simulink model "Ejercicio_Valvulas_simuslx"  (R2021a)
settings: Solver=VariableStepAuto  StartTime=0.0  StopTime=20  RelTol=1e-3
values from neighbouring files (symbols this model uses):
  K = [p1-a1 p2-a2] * Wrm * inv(Wr)    [Controlabilidad.m]    (also in Ejemplo_filminas.m; Ejercicio_Inestable.m = [p1 - a1, p2 - a2] * Wrm * inv(Wr); Ejercicio_Valvulas.m = Ka(1:order(P)); realimentacion_ee.m = acker(A, B, [-10 -10]))
  ue = x3e    [Ejercicio_Valvulas.m]
  xe = [x1e; x2e; x3e]    [Ejercicio_Valvulas.m]
  ye = x1e    (= 2)    [Ejercicio_Valvulas.m]
settings Model: Creator=Santiago  LastModifiedBy=Santiago

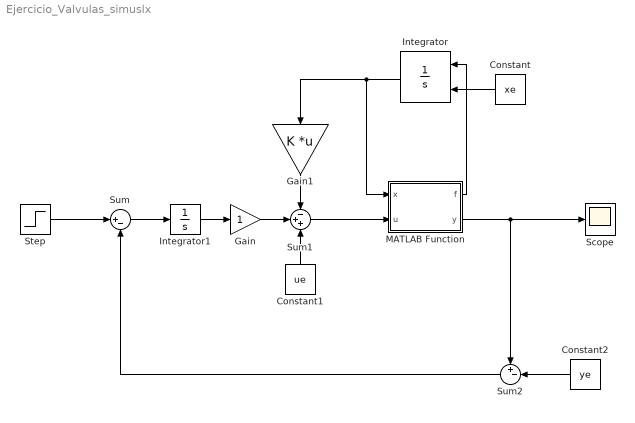
== system Ejercicio_Valvulas_simuslx ==
  Constant : Constant  Value=xe
  Constant1 : Constant  Value=ue
  Constant2 : Constant  Value=ye
  Gain : Gain
  Gain1 : Gain  Gain=K  Multiplication=Matrix(K*u) (u vector)
  Integrator : Integrator  InitialConditionSource=external
  Integrator1 : Integrator
  MATLAB Function : MATLAB Function  TreatAsAtomicUnit=on
  Scope : Scope
  Step : Step  After=0.5  SampleTime=0
  Sum : Sum  Inputs=|+-
  Sum1 : Sum  Inputs=-++
  Sum2 : Sum  Inputs=+-|
  wires:
  MATLAB Function/1(f) -> Integrator/1
  Integrator/1 -> Gain1/1, MATLAB Function/1(x)
  Constant/1 -> Integrator/2
  Gain1/1 -> Sum1/1
  Gain/1 -> Sum1/2
  Integrator1/1 -> Gain/1
  Sum/1 -> Integrator1/1
  Constant1/1 -> Sum1/3
  Sum1/1 -> MATLAB Function/2(u)
  Sum2/1 -> Sum/2
  MATLAB Function/2(y) -> Scope/1, Sum2/1
  Constant2/1 -> Sum2/2
  Step/1 -> Sum/1

== matlab function Ejercicio_Valvulas_simuslx/MATLAB Function ==
  data: x input; f output; u input; y output
function [f, y] = fcn(x, u)
x1 = x(1);
x2 = x(2);
x3 = x(3);
f1 = - sqrt(x1 - x2) + 5 * 40^(x3 - 1);
f2 = sqrt(x1 - x2) - sqrt(x2);
f3 = -x3 + u;
f = [f1; f2; f3];

y = x1;
